simulink model "Adelantamientov_COMPLETO"  (R2020a)
settings: Solver=FixedStepDiscrete  StartTime=0.0  StopTime=45  RelTol=1e-3
model workspace (MAT data in the model file):
  firstWarning = 1
  originalScenarioChecksum = '158070AB835E3E5B039703679FDCB6FF'
values from neighbouring files (symbols this model uses):
  Cd = 0.33    [initialize.m]
  densidadAire = 1.202    [initialize.m]
  fault_d = 200    [initialize.m]
  frontalArea = 1.873    [initialize.m]
  FV2 = 0    [initialize.m]
  FV3 = 0    [initialize.m]
  Fx0 = 0.015*masa*9.81 + 0.5*densidadAire*frontalArea*Cd*(u0+uw)^2    (= 443.33030625)    [initialize.m]
  IV2 = 0    [initialize.m]
  IV3 = 0    [initialize.m]
  masa = 1435    [initialize.m]
  P_ego_init = -200    [initialize.m]
  T2 = 10    [initialize.m]
  T3 = 10    [initialize.m]
  t_gap = 1.5    [initialize.m]
  V_ego_init = 90/3.6    (= 25)    [initialize.m]
undefined symbols (not defined in the file or in its folder): accsubsystem_data, DiscIntNeverNeededParam, driving
libraries: drivingscenarioandsensors x3, drivinglib x2, simulink_extras x2, mpclib x1, mpcadaslib x1
settings Model: Creator=Sun Tzu  LastModifiedBy=derpb

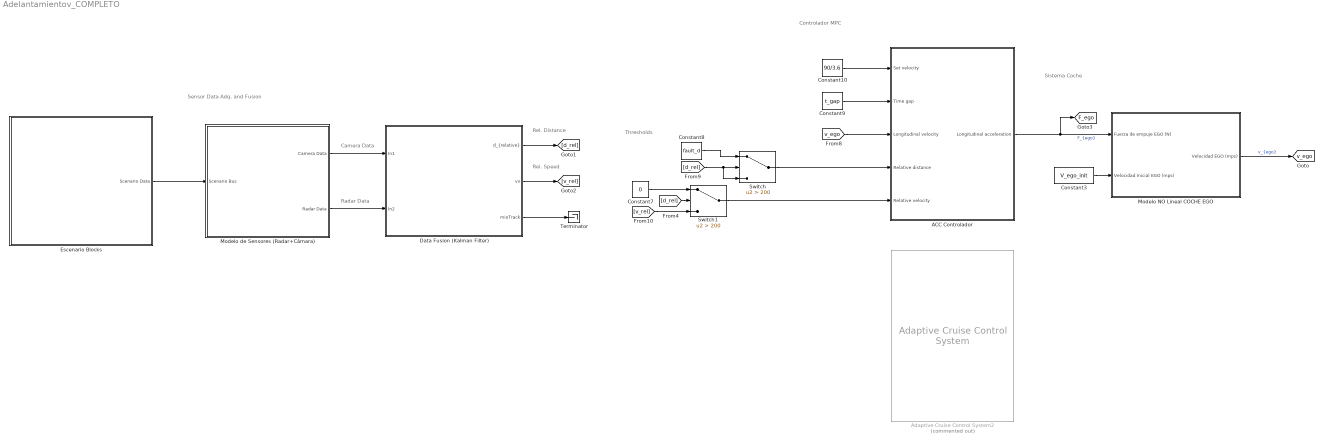
== system Adelantamientov_COMPLETO ==
  note: Camera Data
  note: Sensor Data Adq. and Fusion
  note: Sistema Coche
  note: Controlador MPC
  note: Thresholds
  note: Radar Data
  note: Rel. Distance
  note: Rel. Speed
  ACC Controlador : Subsystem
  Adaptive Cruise Control System2 : mpcadaslib/Adaptive Cruise Control System  Commented=on  EgoModel=tf(0.05,[81.1,1])  InitialEgoVelocity=V_ego_init  DefaultSpacing=10  MaxVelocity=120/3.6  MinAcceleration=Ft_min  amin_ext=off  MaxAcceleration=Ft_max  amax_ext=off  Ts=0.1  PredictionHorizon=30  ControllerBehavior=0.730  suboptimal=off  maxiter=10  datatypeopt=double  optmode=off  trackmode=off
  Constant10 : Constant  Value=90/3.6
  Constant3 : Constant  Value=V_ego_init
  Constant7 : Constant  Value=0
  Constant8 : Constant  Value=fault_d
  Constant9 : Constant  Value=t_gap
  Data Fusion (Kalman Filter) : Subsystem
      mask Display: image('Sensor_Fusion_IMG.png'); % Use "Edit Image" on toolstrip to change.
  Escenario Blocks : Subsystem
      mask Display: image('Scenario_IMG.JPG'); % Use "Edit Image" on toolstrip to change.
  Modelo NO Lineal COCHE EGO : Subsystem
  Modelo de Sensores (Radar+Cámara) : Subsystem
      mask Display: image('Captura.JPG'); % Use "Edit Image" on toolstrip to change.
  Switch : Switch  Criteria=u2 > Threshold  Threshold=200
  Switch1 : Switch  Criteria=u2 > Threshold  Threshold=200
  Terminator : Terminator
  tag scope: F_ego=global, v_ego=global
  wires:
  Constant8/1 -> Switch/1
  Switch/1 -> ACC Controlador/4(Relative distance)
  [d_rel] -> Switch1/2
  Constant7/1 -> Switch1/1
  [v_rel] -> Switch1/3
  [d_rel] -> Switch/3, Switch/2
  Switch1/1 -> ACC Controlador/5(Relative velocity)
  [v_ego] -> ACC Controlador/3(Longitudinal velocity)
  ACC Controlador/1(Longitudinal acceleration) -> [F_ego], Modelo NO Lineal COCHE EGO/1(Fuerza de empuje EGO (N))  "F_{ego}"
  Constant10/1 -> ACC Controlador/1(Set velocity)
  Constant9/1 -> ACC Controlador/2(Time gap)
  Modelo NO Lineal COCHE EGO/1(Velocidad EGO (mps)) -> [v_ego]  "v_{ego}"
  Constant3/1 -> Modelo NO Lineal COCHE EGO/2(Velocidad Inicial EGO (mps))
  Escenario Blocks/1(Scenario Data) -> Modelo de Sensores (Radar+Cámara)/1(Scenario Bus)
  Data Fusion (Kalman Filter)/1("d_{relative}") -> [d_rel]
  Data Fusion (Kalman Filter)/2(vx) -> [v_rel]
  Modelo de Sensores (Radar+Cámara)/1(Camera Data) -> Data Fusion (Kalman Filter)/1(In1)
  Modelo de Sensores (Radar+Cámara)/2(Radar Data) -> Data Fusion (Kalman Filter)/2(In2)
  Data Fusion (Kalman Filter)/3(mioTrack) -> Terminator/1

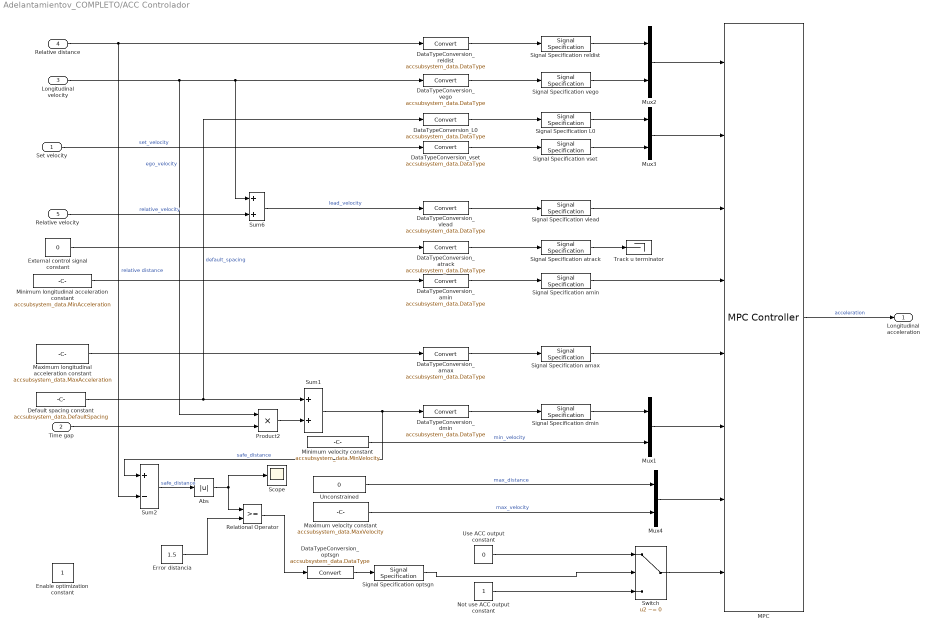
== system Adelantamientov_COMPLETO/ACC Controlador ==
  Set velocity : Inport
  Time gap : Inport  Port=2
  Longitudinal velocity : Inport  Port=3
  Relative distance : Inport  Port=4
  Relative velocity : Inport  Port=5
  Abs : Abs
  DataTypeConversion_L0 : DataTypeConversion  OutDataTypeStr=accsubsystem_data.DataType
  DataTypeConversion_amax : DataTypeConversion  OutDataTypeStr=accsubsystem_data.DataType
  DataTypeConversion_amin : DataTypeConversion  OutDataTypeStr=accsubsystem_data.DataType
  DataTypeConversion_atrack : DataTypeConversion  OutDataTypeStr=accsubsystem_data.DataType
  DataTypeConversion_dmin : DataTypeConversion  OutDataTypeStr=accsubsystem_data.DataType
  DataTypeConversion_optsgn : DataTypeConversion  OutDataTypeStr=accsubsystem_data.DataType
  DataTypeConversion_reldist : DataTypeConversion  OutDataTypeStr=accsubsystem_data.DataType
  DataTypeConversion_vego : DataTypeConversion  OutDataTypeStr=accsubsystem_data.DataType
  DataTypeConversion_vlead : DataTypeConversion  OutDataTypeStr=accsubsystem_data.DataType
  DataTypeConversion_vset : DataTypeConversion  OutDataTypeStr=accsubsystem_data.DataType
  Default spacing constant : Constant  Value=accsubsystem_data.DefaultSpacing  OutDataTypeStr=accsubsystem_data.DataType
  Enable optimization constant : Constant  OutDataTypeStr=accsubsystem_data.DataType
  Error distancia : Constant  Value=1.5  OutDataTypeStr=accsubsystem_data.DataType
  External control signal constant : Constant  Value=0  OutDataTypeStr=accsubsystem_data.DataType
  MPC : mpclib/MPC Controller  SCDEnableBlockLinearizationSpecification=on  mpcobj=accsubsystem_data.Controller  is_multiple=0  enable_value=0  return_u0=off  updateMPCinCallerWorkspace=off  md_inport=on  mv_inport=off  uref_inport=off  return_cost=off  return_mvseq=off  return_qpstatus=off  return_xseq=off  return_state=off  return_ovseq=off  state_inport=off  umin_inport=on  umax_inport=on  ymin_inport=on  ymax_inport=on  cc_inport=off  ywt_inport=off  uwt_inport=off  duwt_inport=off  rhoeps_inport=off  pm_inport=off  MaximumP=10  HorizonChoice=FixedHorizon  n_ts=0.1  n_p=30  n_mv=1  n_md=1  n_ud=0  n_mo=2  n_uo=0  BlockDataType=double  SampleTimeInherited=off  switch_inport=on
  Maximum longitudinal acceleration constant : Constant  Value=accsubsystem_data.MaxAcceleration  OutDataTypeStr=accsubsystem_data.DataType
  Maximum velocity constant : Constant  Value=accsubsystem_data.MaxVelocity  OutDataTypeStr=accsubsystem_data.DataType
  Minimum longitudinal acceleration constant : Constant  Value=accsubsystem_data.MinAcceleration  OutDataTypeStr=accsubsystem_data.DataType
  Minimum velocity constant : Constant  Value=accsubsystem_data.MinVelocity  OutDataTypeStr=accsubsystem_data.DataType
  Mux{1..4} (4 alike) : Mux  Inputs=[1 1]
  Not use ACC output constant : Constant  OutDataTypeStr=accsubsystem_data.DataType
  Product2 : Product
  Relational Operator : RelationalOperator  OutDataTypeStr=boolean  RndMeth=Simplest
  Scope : Scope
  Signal Specification L0 : SignalSpecification  Dimensions=1
  Signal Specification amax : SignalSpecification  Dimensions=1
  Signal Specification amin : SignalSpecification  Dimensions=1
  Signal Specification atrack : SignalSpecification  Dimensions=1
  Signal Specification dmin : SignalSpecification  Dimensions=1
  Signal Specification optsgn : SignalSpecification  Dimensions=1
  Signal Specification reldist : SignalSpecification  Dimensions=1
  Signal Specification vego : SignalSpecification  Dimensions=1
  Signal Specification vlead : SignalSpecification  Dimensions=1
  Signal Specification vset : SignalSpecification  Dimensions=1
  Sum1 : Sum
  Sum2 : Sum  Inputs=+-
  Sum6 : Sum
  Switch : Switch  Criteria=u2 ~= 0
  Track u terminator : Terminator
  Unconstrained : Constant  Value=0  OutDataTypeStr=accsubsystem_data.DataType
  Use ACC output constant : Constant  Value=0  OutDataTypeStr=accsubsystem_data.DataType
  Longitudinal acceleration : Outport  PortDimensions=1  VectorParamsAs1DForOutWhenUnconnected=off
  wires:
  Sum6/1 -> DataTypeConversion_vlead/1  "lead_velocity"
  Default spacing constant/1 -> DataTypeConversion_L0/1, Sum1/1  "default_spacing"
  Mux2/1 -> MPC/1
  Mux3/1 -> MPC/2
  Longitudinal velocity/1 -> Product2/1, DataTypeConversion_vego/1, Sum6/1  "ego_velocity"
  Relative distance/1 -> DataTypeConversion_reldist/1, Sum2/2  "relative distance"
  Relative velocity/1 -> Sum6/2  "relative_velocity"
  MPC/1 -> Longitudinal acceleration/1  "acceleration"
  Product2/1 -> Sum1/2
  Minimum velocity constant/1 -> Mux1/2  "min_velocity"
  Sum1/1 -> Sum2/1, DataTypeConversion_dmin/1  "safe_distance"
  DataTypeConversion_amax/1 -> Signal Specification amax/1
  DataTypeConversion_amin/1 -> Signal Specification amin/1
  DataTypeConversion_atrack/1 -> Signal Specification atrack/1
  Mux1/1 -> MPC/6
  Signal Specification amax/1 -> MPC/5
  Signal Specification amin/1 -> MPC/4
  Switch/1 -> MPC/8
  Use ACC output constant/1 -> Switch/1
  Not use ACC output constant/1 -> Switch/3
  DataTypeConversion_dmin/1 -> Signal Specification dmin/1
  Signal Specification dmin/1 -> Mux1/1
  DataTypeConversion_vlead/1 -> Signal Specification vlead/1
  Signal Specification vlead/1 -> MPC/3
  DataTypeConversion_L0/1 -> Signal Specification L0/1
  Signal Specification L0/1 -> Mux3/1
  DataTypeConversion_vset/1 -> Signal Specification vset/1
  Signal Specification vset/1 -> Mux3/2
  DataTypeConversion_reldist/1 -> Signal Specification reldist/1
  Signal Specification reldist/1 -> Mux2/1
  DataTypeConversion_vego/1 -> Signal Specification vego/1
  Signal Specification vego/1 -> Mux2/2
  Time gap/1 -> Product2/2
  Set velocity/1 -> DataTypeConversion_vset/1  "set_velocity"
  DataTypeConversion_optsgn/1 -> Signal Specification optsgn/1
  Signal Specification optsgn/1 -> Switch/2
  Signal Specification atrack/1 -> Track u terminator/1
  External control signal constant/1 -> DataTypeConversion_atrack/1
  Minimum longitudinal acceleration constant/1 -> DataTypeConversion_amin/1
  Maximum longitudinal acceleration constant/1 -> DataTypeConversion_amax/1
  Mux4/1 -> MPC/7
  Maximum velocity constant/1 -> Mux4/2  "max_velocity"
  Unconstrained/1 -> Mux4/1  "max_distance"
  Error distancia/1 -> Relational Operator/2
  Abs/1 -> Scope/1, Relational Operator/1
  Sum2/1 -> Abs/1  "safe_distance"
  Relational Operator/1 -> DataTypeConversion_optsgn/1

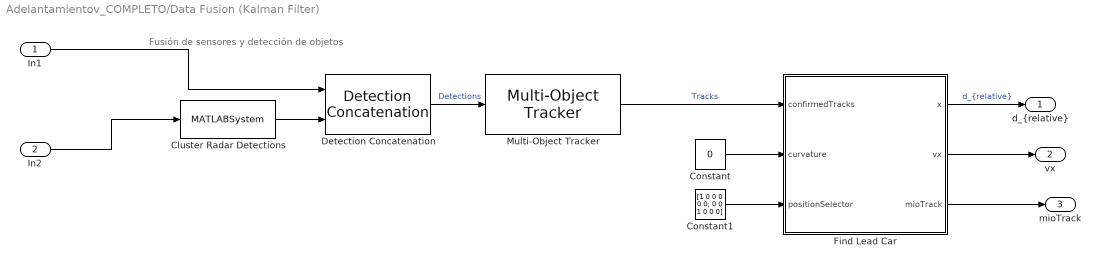
== system Adelantamientov_COMPLETO/Data Fusion (Kalman Filter) ==
  note: Fusión de sensores y detección de objetos
  In1 : Inport
  In2 : Inport  Port=2
  Cluster Radar Detections : MATLABSystem  System=helperClusterDetections  ClusterSize=5  BusNameSource=Auto  BusName=BusClusterDetections  SimulateUsing=Interpreted execution
      mask Type: helperClusterDetections
      mask Display:
      | disp(['Detection' char(10) 'Clustering']);
      | port_label('input',1,'In');
      | port_label('output',1,'Out');
  Constant : Constant  Value=0
  Constant1 : Constant  Value=[1 0 0 0 0 0; 0 0 1 0 0 0]
  Detection Concatenation : drivinglib/Detection Concatenation  NumInputs=2  BusNameSource=Auto  BusName=BusDetectionConcatenation1  SimulateUsing=Interpreted execution
      settings: SourceProductBaseCode=DR
  Find Lead Car : MATLAB Function  TreatAsAtomicUnit=on
  Multi-Object Tracker : drivinglib/Multi-Object Tracker  TrackerIndex=uint32( 0 )  FilterInitializationFcn=helperInitSimulinkDemoFilter  AssignmentThreshold=50  ConfirmationThreshold=[ 2, 3 ]  DeletionThreshold=[ 5, 5 ]  MaxNumTracks=20  MaxNumSensors=8  StateParams=struct  TimeInputSource=Auto  HasCostMatrixInput=off  HasDetectableTrackIDsInput=off  BusNameSource=Auto  BusName=BusMultiObjectTracker1  TentativeTracksOutputPort=off  AllTracksOutputPort=off  SimulateUsing=Interpreted execution
      settings: SourceProductBaseCode=DR
  "d_{relative}" : Outport
  vx : Outport  Port=2
  mioTrack : Outport  Port=3
  wires:
  In1/1 -> Detection Concatenation/1
  Cluster Radar Detections/1 -> Detection Concatenation/2
  Detection Concatenation/1 -> Multi-Object Tracker/1  "Detections"
  Constant1/1 -> Find Lead Car/3(positionSelector)
  Find Lead Car/3(mioTrack) -> mioTrack/1
  Multi-Object Tracker/1 -> Find Lead Car/1(confirmedTracks)  "Tracks"
  Find Lead Car/2(vx) -> vx/1
  Constant/1 -> Find Lead Car/2(curvature)
  Find Lead Car/1(x) -> "d_{relative}"/1  "d_{relative}"
  In2/1 -> Cluster Radar Detections/1

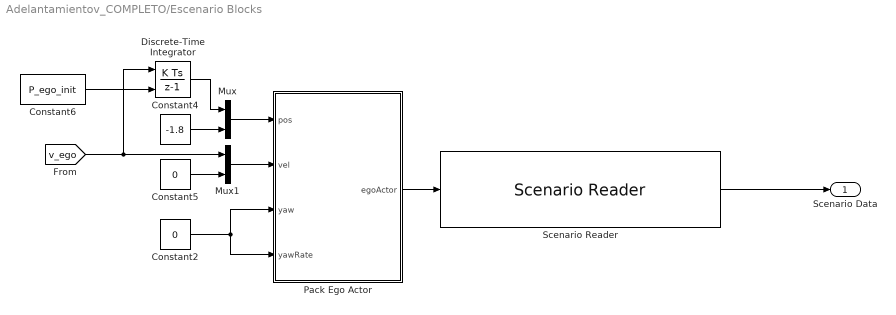
== system Adelantamientov_COMPLETO/Escenario Blocks ==
  Constant2 : Constant  Value=0
  Constant4 : Constant  Value=-1.8
  Constant5 : Constant  Value=0
  Constant6 : Constant  Value=P_ego_init
  Discrete-Time Integrator : DiscreteIntegrator  InitialConditionSource=external  InitialCondition=5  SampleTime=-1  ICPrevOutput=DiscIntNeverNeededParam  ICPrevScaledInput=DiscIntNeverNeededParam
  Mux : Mux  Inputs=2
  Mux1 : Mux  Inputs=2
  Pack Ego Actor : MATLAB Function  TreatAsAtomicUnit=on
  Scenario Reader : drivingscenarioandsensors/Scenario Reader  ScenarioSource=From file  ScenarioFileName=EscenarioAdelantamientov5.mat  ScenarioVariableName=scenario  OutputCoordinateSystem=Vehicle coordinates  EgoVehicleSource=Input port  OrientVehiclesOnRoad=off  EgoVehicleActorID=1  OutputEgoVehiclePose=off  SampleTime=0.1  LaneBoundaryOutput=None  LaneBoundaryDistance=0:0.5:9.5  LaneBoundaryLocation=Center of lane markings  BusNameSource=Auto  BusName=BusActorsActors  BusName2Source=Auto  BusName2=BusLaneBoundaries  BusName3Source=Auto  BusName3=BusEgoActor  ShowCoordinateLabels=on  SimulateUsing=Interpreted execution
  Scenario Data : Outport
  wires:
  Constant6/1 -> Discrete-Time Integrator/2
  [v_ego] -> Discrete-Time Integrator/1, Mux1/1
  Constant4/1 -> Mux/2
  Mux/1 -> Pack Ego Actor/1(pos)
  Mux1/1 -> Pack Ego Actor/2(vel)
  Pack Ego Actor/1(egoActor) -> Scenario Reader/1
  Discrete-Time Integrator/1 -> Mux/1
  Constant2/1 -> Pack Ego Actor/4(yawRate), Pack Ego Actor/3(yaw)
  Constant5/1 -> Mux1/2
  Scenario Reader/1 -> Scenario Data/1

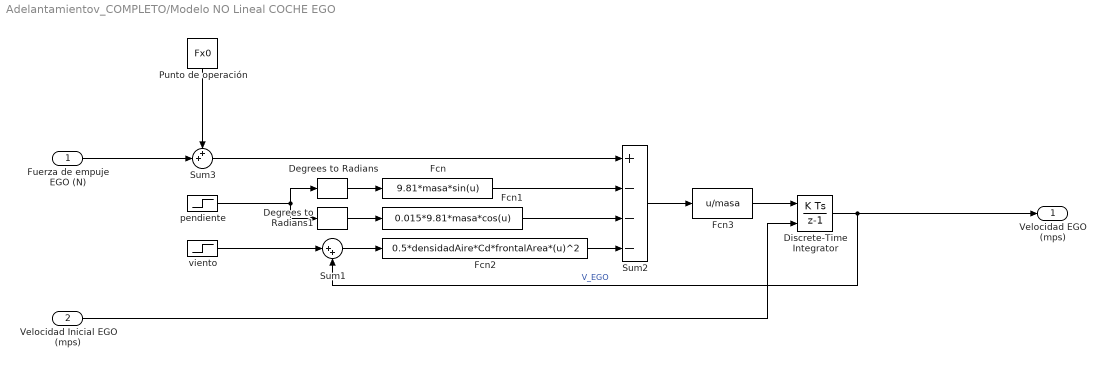
== system Adelantamientov_COMPLETO/Modelo NO Lineal COCHE EGO ==
  Fuerza de empuje EGO (N) : Inport
  Velocidad Inicial EGO (mps) : Inport  Port=2
  Degrees to Radians : simulink_extras/Transformations/Degrees to Radians
  Degrees to Radians1 : simulink_extras/Transformations/Degrees to Radians
  Discrete-Time Integrator : DiscreteIntegrator  InitialConditionSource=external  SampleTime=-1  ICPrevOutput=DiscIntNeverNeededParam  ICPrevScaledInput=DiscIntNeverNeededParam
  Fcn : Fcn  Expr=9.81*masa*sin(u)
  Fcn1 : Fcn  Expr=0.015*9.81*masa*cos(u)
  Fcn2 : Fcn  Expr=0.5*densidadAire*Cd*frontalArea*(u)^2
  Fcn3 : Fcn  Expr=u/masa
  Punto de operación : Constant  Value=Fx0
  Sum1 : Sum  Inputs=|++
  Sum2 : Sum  Inputs=+---
  Sum3 : Sum  Inputs=++|
  pendiente : Step  Time=T2  Before=IV2  After=FV2  SampleTime=0
  viento : Step  Time=T3  Before=IV3  After=FV3  SampleTime=0
  Velocidad EGO (mps) : Outport  VectorParamsAs1DForOutWhenUnconnected=off
  wires:
  Discrete-Time Integrator/1 -> Velocidad EGO (mps)/1, Sum1/2  "V_EGO"
  Velocidad Inicial EGO (mps)/1 -> Discrete-Time Integrator/2
  Punto de operación/1 -> Sum3/1
  Fuerza de empuje EGO (N)/1 -> Sum3/2
  Sum3/1 -> Sum2/1
  viento/1 -> Sum1/1
  Sum1/1 -> Fcn2/1
  Fcn1/1 -> Sum2/3
  Degrees to Radians1/1 -> Fcn1/1
  Fcn3/1 -> Discrete-Time Integrator/1
  Fcn/1 -> Sum2/2
  pendiente/1 -> Degrees to Radians/1, Degrees to Radians1/1
  Degrees to Radians/1 -> Fcn/1
  Sum2/1 -> Fcn3/1
  Fcn2/1 -> Sum2/4

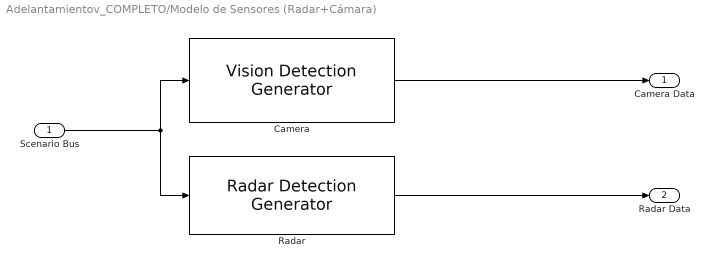
== system Adelantamientov_COMPLETO/Modelo de Sensores (Radar+Cámara) ==
  Scenario Bus : Inport
  Camera : drivingscenarioandsensors/Vision Detection Generator  SensorIndex=1  DetectorOutput=Objects only  UpdateInterval=0.1  LaneUpdateInterval=0.1  SensorLocation=[1.9 0]  Height=1.1  Yaw=0  Pitch=1  Roll=0  BusNameSource=Auto  BusName=BusObjectDetections  BusName2Source=Auto  BusName2=BusLaneDetections  MaxNumDetectionsSource=Property  MaxNumDetections=50  MaxNumLanesSource=Property  MaxNumLanes=30  DetectionCoordinates=Ego Cartesian  SimulateUsing=Interpreted execution  MaxRange=100  BoundingBoxAccuracy=5  ProcessNoiseIntensity=5  MaxSpeed=50  MaxAllowedOcclusion=0.5  MinObjectImageSize=[15 15]  DetectionProbability=0.9  FalsePositivesPerImage=0.1  MinLaneImageSize=[20 3]  LaneBoundaryAccuracy=3  HasNoise=on  InitialSeedSource=Repeatable  InitialSeed=0  UsedSeed=0  ActorProfilesSource=MATLAB expression  ActorProfilesParameters=driving.internal.ActorProfilesParameters  ActorProfilesExpression=[struct('ActorID',1,'ClassID',6,'Length',4.7,'Width',1.8,'Height',1.4,'OriginOffset',[-1.35 0 0],'RCSPattern',[10 10;10 10],'RCSAzimuthAngles',[-180 180],'RCSElevationAngles',[-90 90]); struct('ActorID',2,'ClassID',2,'Length',8.2,'Width',2.5,'Height',3.5,'OriginOffset',[-3.1 0 0],'RCSPattern',[10 10;10 10],'RCSAzimuthAngles',[-180 180],'RCSElevationAngles',[-90 90]); struct('ActorID',3,'ClassID',2,'Length',8.2,'Width',2.5,'Height',3.5,'OriginOffset',[-3.1 0 0],'RCSPattern',[10 10;10 10],'RCSAzimuthAngles',[-180 180],'RCSElevationAngles',[-90 90]); struct('ActorID',4,'ClassID',1,'Length',4.7,'Width',1.8,'Height',1.4,'OriginOffset',[-1.35 0 0],'RCSPattern',[10 10;10 10],'RCSAzimuthAngles',[-180 180],'RCSElevationAngles',[-90 90])]  Intrinsics=driving.internal.cameraIntrinsics('FocalLength',[1814.81018227767 1814.81018227767],'PrincipalPoint',[320 240],'ImageSize',[480 640],'RadialDistortion',[0 0],'TangentialDistortion',[0 0],'Skew',0)
  Radar : drivingscenarioandsensors/Radar Detection Generator  SensorIndex=2  UpdateInterval=0.1  SensorLocation=[3.7 0]  Height=0.2  Yaw=0  Pitch=0  Roll=0  BusNameSource=Auto  BusName=BusRadarDetectionGenerator  MaxNumDetectionsSource=Property  MaxNumDetections=50  DetectionCoordinates=Ego Cartesian  SimulateUsing=Interpreted execution  AzimuthResolution=4  ElevationResolution=10  RangeResolution=2.5  RangeRateResolution=0.5  AzimuthBiasFraction=0.1  ElevationBiasFraction=0.1  RangeBiasFraction=0.05  RangeRateBiasFraction=0.05  FieldOfView=[10 5]  MaxRange=200  RangeRateLimits=[-100 100]  DetectionProbability=0.9  FalseAlarmRate=1e-06  ReferenceRange=150  ReferenceRCS=0  HasElevation=off  HasRangeRate=on  HasNoise=on  HasFalseAlarms=on  HasOcclusion=on  InitialSeedSource=Repeatable  InitialSeed=0  UsedSeed=0  ActorProfilesSource=MATLAB expression  ActorProfilesParameters=driving.internal.ActorProfilesRadarParameters  ActorProfilesExpression=[struct('ActorID',1,'ClassID',6,'Length',4.7,'Width',1.8,'Height',1.4,'OriginOffset',[-1.35 0 0],'RCSPattern',[10 10;10 10],'RCSAzimuthAngles',[-180 180],'RCSElevationAngles',[-90 90]); struct('ActorID',2,'ClassID',2,'Length',8.2,'Width',2.5,'Height',3.5,'OriginOffset',[-3.1 0 0],'RCSPattern',[10 10;10 10],'RCSAzimuthAngles',[-180 180],'RCSElevationAngles',[-90 90]); struct('ActorID',3,'ClassID',2,'Length',8.2,'Width',2.5,'Height',3.5,'OriginOffset',[-3.1 0 0],'RCSPattern',[10 10;10 10],'RCSAzimuthAngles',[-180 180],'RCSElevationAngles',[-90 90]); struct('ActorID',4,'ClassID',1,'Length',4.7,'Width',1.8,'Height',1.4,'OriginOffset',[-1.35 0 0],'RCSPattern',[10 10;10 10],'RCSAzimuthAngles',[-180 180],'RCSElevationAngles',[-90 90])]
      settings: SourceProductBaseCode=DR
  Camera Data : Outport
  Radar Data : Outport  Port=2
  wires:
  Scenario Bus/1 -> Camera/1, Radar/1
  Radar/1 -> Radar Data/1
  Camera/1 -> Camera Data/1

== matlab function Adelantamientov_COMPLETO/Data Fusion (Kalman Filter)/Find Lead Car ==
  data: confirmedTracks input; x output double size=[1 1]; vx output size=[1 1]; curvature input; mioTrack output; positionSelector input
function [x,vx,mioTrack] = findLeadCar(confirmedTracks, curvature, positionSelector)
% This function finds the lead car: a car in front of the ego car that
% satisfies all the criteria below:
% * Within the ego car's lane.
% * In front of the ego car.
% * Closest to the ego car.

% Important notes:
% 1. If you change state definition, change the following:
%       State = [x;vx;y;vy;z;vz] (3D constant velocity)
numStates = 6;

% 2. The lane is defined using a parabolic model, where y=ax^2+bx+c. a is
%    equal to half the road curvature, b=0, and c is the offset of the lane
%    boundaries relative to the ego car. Overall lane width is assumed to
%    be 3.6m, typical highway lane width.
laneWidth = 3.6;

% 3. The ego car is assumed to be traveling in the middle of its lane, with
%    1.8m on each side of it. So, c=+1.8m for the left lane boundary and
%    -1.8m for the right lane boundary.
halfLaneWidth = laneWidth/2;

% Initialize outputs and parameters
maxX = cast(1000, 'like', confirmedTracks.Tracks(1).State);  % Far enough forward so that no track is expected to exceed this distance
trackID = 0;

for i = 1:confirmedTracks.NumTracks
    position = positionSelector * confirmedTracks.Tracks(i).State;
    x = position(1); % Longitudinal position of the track relative to ego
    y = position(2); % Lateral position of the track relative to ego
    
    if x < maxX && x > 0 % No point checking otherwise
        yleftLane  = polyval([curvature/2, 0,  halfLaneWidth],x); % Half a lane to the left
        yrightLane = polyval([curvature/2, 0, -halfLaneWidth],x); % Half a lane to the right
        
        % Find a new lead car
        if (yrightLane <= y) && (y <= yleftLane)
            maxX = x;
            trackID = i;
        end
    end
end

if trackID>0
    mioState = confirmedTracks.Tracks(trackID).State;
else
    mioState = inf(numStates,1,'like',confirmedTracks.Tracks(1).State);
end

% Output:
x = mioState(1);    % Longitudinal position of the lead car
vx = mioState(2);   % Longitudinal velocity of the lead car
mioTrack = trackID; % Index of the most important track

== matlab function Adelantamientov_COMPLETO/Escenario Blocks/Pack Ego Actor ==
  data: pos input; egoActor output Bus: BusActors1Actors size=1; vel input; yaw input; yawRate input
function egoActor = packEgo(pos,vel,yaw,yawRate)
% Pack ego information into a single ego actor bus
%
% Imoprtant note:
% Output is a bus of type BusActorsActors. This is the same bus used by the
% Scenario Reader to output an individual actor. If you change the
% output bus name of Scenario Reader, change the output bus name here
% as well by clicking on 'Edit Data' in the menu above.

egoActor = struct(...
    'ActorID',1,...
    'Position', [pos(1) pos(2) 0], ...
    'Velocity', [vel(1) vel(2) 0], ...
    'Roll', 0, ...
    'Pitch', 0, ...
    'Yaw', yaw, ...
    'AngularVelocity', [0 0 yawRate]);
